simulink model "microgrid3"  (R2020a)
settings: Solver=VariableStepAuto  StartTime=0.0  StopTime=14.4  RelTol=1e-3
model workspace (MAT data in the model file):
  Sig = Simulink.Signal
  Sig.DataType = 'auto'
  Sig.Dimensions = -1
  Sig.DimensionsMode = 'auto'
  Sig.Complexity = 'auto'
  Sig.SampleTime = -1
  Sig.SamplingMode = 'auto'
libraries: powerlib x76, powerlib_meascontrol x32, eePowerMeasurement x10
settings Model: OrderedModelArguments=off  Creator=ramaz  LastModifiedBy=ramaz

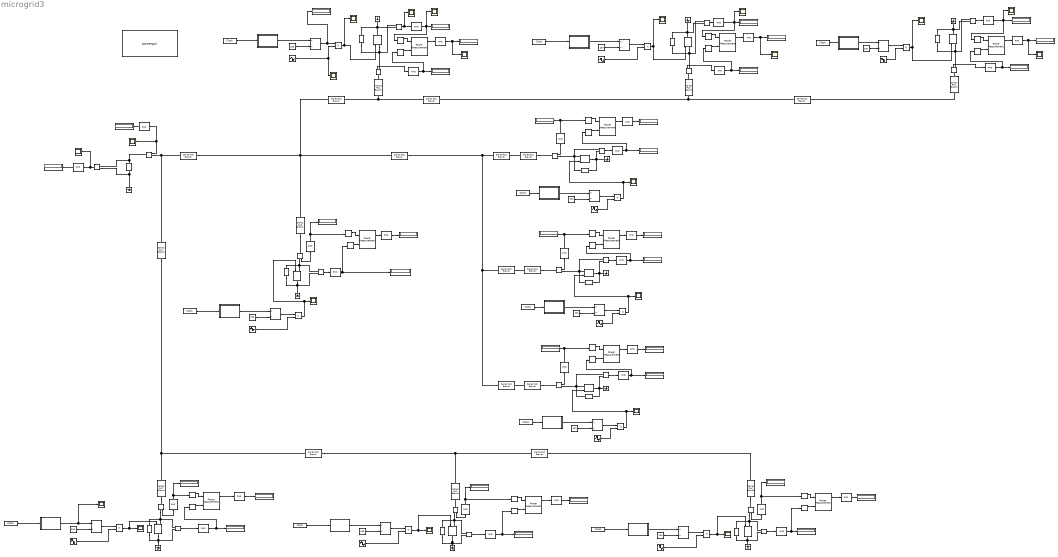
== system microgrid3 ==
  AC Voltage Source : powerlib/Electrical Sources/AC Voltage Source  Amplitude=325  Phase=0  Frequency=50  SampleTime=0  Measurements=Voltage  BusType=swing  Pref=10e3  Qref=0  Qmin=-inf  Qmax=+inf
  AMKA 16 - 45m : powerlib/Elements/Series RLC Branch  LConnTagsString=__new0  RConnTagsString=__new0  BranchType=RL  Resistance=0.08595  Inductance=1.5469860468e-5  SetiL0=off  InitialCurrent=0  Capacitance=1e-6  Setx0=off  InitialVoltage=0  Measurements=None
  AMKA 25 - 58m : powerlib/Elements/Series RLC Branch  LConnTagsString=__new0  RConnTagsString=__new0  BranchType=RL  Resistance=0.0696  Inductance=1.9569691802e-5  SetiL0=off  InitialCurrent=0  Capacitance=1e-6  Setx0=off  InitialVoltage=0  Measurements=None
  AMKA 35 - 137m : powerlib/Elements/Series RLC Branch  LConnTagsString=__new0  RConnTagsString=__new0  BranchType=RL  Resistance=0.087817  Inductance=4.4044538951e-5  SetiL0=off  InitialCurrent=0  Capacitance=1e-6  Setx0=off  InitialVoltage=0  Measurements=None
  AMKA 35 - 248m : powerlib/Elements/Series RLC Branch  LConnTagsString=__new0  RConnTagsString=__new0  BranchType=RL  Resistance=0.158968  Inductance=7.9730260291e-5  SetiL0=off  InitialCurrent=0  Capacitance=1e-6  Setx0=off  InitialVoltage=0  Measurements=None
  AMKA 35 - 33m : powerlib/Elements/Series RLC Branch  LConnTagsString=__new0  RConnTagsString=__new0  BranchType=RL  Resistance=0.021153  Inductance=1.0609268506e-5  SetiL0=off  InitialCurrent=0  Capacitance=1e-6  Setx0=off  InitialVoltage=0  Measurements=None
  AMKA 35 - 52m : powerlib/Elements/Series RLC Branch  LConnTagsString=__new0  RConnTagsString=__new0  BranchType=RL  Resistance=0.033332  Inductance=1.6717635222e-5  SetiL0=off  InitialCurrent=0  Capacitance=1e-6  Setx0=off  InitialVoltage=0  Measurements=None
  AMKA 35 - 85m : powerlib/Elements/Series RLC Branch  LConnTagsString=__new0  RConnTagsString=__new0  BranchType=RL  Resistance=0.054485  Inductance=2.8612875669e-5  SetiL0=off  InitialCurrent=0  Capacitance=1e-6  Setx0=off  InitialVoltage=0  Measurements=None
  AMKA 35 - 89m : powerlib/Elements/Series RLC Branch  LConnTagsString=__new0  RConnTagsString=__new0  BranchType=RL  Resistance=0.057049  Inductance=2.8612875669e-5  SetiL0=off  InitialCurrent=0  Capacitance=1e-6  Setx0=off  InitialVoltage=0  Measurements=None
  AMKA 35 - 95m : powerlib/Elements/Series RLC Branch  LConnTagsString=__new0  RConnTagsString=__new0  BranchType=RL  Resistance=0.060895  Inductance=3.0541833579e-5  SetiL0=off  InitialCurrent=0  Capacitance=1e-6  Setx0=off  InitialVoltage=0  Measurements=None
  AMKA 35 -89m : powerlib/Elements/Series RLC Branch  LConnTagsString=__new0  RConnTagsString=__new0  BranchType=RL  Resistance=0.03846  Inductance=1.9289579102e-5  SetiL0=off  InitialCurrent=0  Capacitance=1e-6  Setx0=off  InitialVoltage=0  Measurements=None
  AXMK 50 - 571m : powerlib/Elements/Series RLC Branch  LConnTagsString=__new0  RConnTagsString=__new0  BranchType=RL  Resistance=0.366011  Inductance=0.000159944351  SetiL0=off  InitialCurrent=0  Capacitance=1e-6  Setx0=off  InitialVoltage=0  Measurements=None
  Complex to Real-Imag{1..20} (20 alike) : ComplexToRealImag
  Constant{,1..9} (10 alike) : Constant  Value=230
  Controlled Current Source{1..10} (10 alike) : powerlib/Electrical Sources/Controlled Current Source  Initialize=on  Source_Type=AC  Amplitude=0  Phase=0  Frequency=50  Measurements=None
  Current Display : Display
  Current Display {1..11} (11 alike) : Display
  Current Measurement{,1..6,8..11} (11 alike) : powerlib/Measurements/Current Measurement  PhasorSimulation=off  OutputType=Complex  PSBequivalent=0
  Digital Clock{,1..9} (10 alike) : DigitalClock  SampleTime=0.01
  Divide{,1..9} (10 alike) : Product  Inputs=*/
  Ground{,1..10} (11 alike) : powerlib/Elements/Ground  LConnTagsString=a
  MATLAB Function : MATLAB Function  TreatAsAtomicUnit=on
  MATLAB Function1 : MATLAB Function  TreatAsAtomicUnit=on
  MATLAB Function2 : MATLAB Function  TreatAsAtomicUnit=on
  MATLAB Function3 : MATLAB Function  TreatAsAtomicUnit=on
  MATLAB Function4 : MATLAB Function  TreatAsAtomicUnit=on
  MATLAB Function5 : MATLAB Function  TreatAsAtomicUnit=on
  MATLAB Function6 : MATLAB Function  TreatAsAtomicUnit=on
  MATLAB Function7 : MATLAB Function  TreatAsAtomicUnit=on
  MATLAB Function8 : MATLAB Function  TreatAsAtomicUnit=on
  MATLAB Function9 : MATLAB Function  TreatAsAtomicUnit=on
  MC& - 40m : powerlib/Elements/Series RLC Branch  LConnTagsString=__new0  RConnTagsString=__new0  BranchType=RL  Resistance=0.1232  Inductance=1.1459155902e-5  SetiL0=off  InitialCurrent=0  Capacitance=1e-6  Setx0=off  InitialVoltage=0  Measurements=None
  MC10 - 12m : powerlib/Elements/Series RLC Branch  LConnTagsString=__new0  RConnTagsString=__new0  BranchType=RL  Resistance=0.02196  Inductance=3.3613523981e-6  SetiL0=off  InitialCurrent=0  Capacitance=1e-6  Setx0=off  InitialVoltage=0  Measurements=None
  MC10 - 29m : powerlib/Elements/Series RLC Branch  LConnTagsString=__new0  RConnTagsString=__new0  BranchType=RL  Resistance=0.06954  Inductance=1.0644282593e-6  SetiL0=off  InitialCurrent=0  Capacitance=1e-6  Setx0=off  InitialVoltage=0  Measurements=None
  MC10 - 34m : powerlib/Elements/Series RLC Branch  LConnTagsString=__new0  RConnTagsString=__new0  BranchType=RL  Resistance=0.06222  Inductance=9.5238317946e-6  SetiL0=off  InitialCurrent=0  Capacitance=1e-6  Setx0=off  InitialVoltage=0  Measurements=None
  MC10 - 35m : powerlib/Elements/Series RLC Branch  LConnTagsString=__new0  RConnTagsString=__new0  BranchType=RL  Resistance=0.06405  Inductance=9.803944944e-6  SetiL0=off  InitialCurrent=0  Capacitance=1e-6  Setx0=off  InitialVoltage=0  Measurements=None
  MC10 - 38m : powerlib/Elements/Series RLC Branch  LConnTagsString=__new0  RConnTagsString=__new0  BranchType=RL  Resistance=0.06954  Inductance=1.0644282593e-6  SetiL0=off  InitialCurrent=0  Capacitance=1e-6  Setx0=off  InitialVoltage=0  Measurements=None
  "MC10 - 38m (2) " : powerlib/Elements/Series RLC Branch  LConnTagsString=__new0  RConnTagsString=__new0  BranchType=RL  Resistance=0.06954  Inductance=1.0644282593e-5  SetiL0=off  InitialCurrent=0  Capacitance=1e-6  Setx0=off  InitialVoltage=0  Measurements=None
  MC10 - 48m : powerlib/Elements/Series RLC Branch  LConnTagsString=__new0  RConnTagsString=__new0  BranchType=RL  Resistance=0.08784  Inductance=1.3502705371e-5  SetiL0=off  InitialCurrent=0  Capacitance=1e-6  Setx0=off  InitialVoltage=0  Measurements=None
  MC6 - 11m : powerlib/Elements/Series RLC Branch  LConnTagsString=__new0  RConnTagsString=__new0  BranchType=RL  Resistance=0.03388  Inductance=3.1512678737e-6  SetiL0=off  InitialCurrent=0  Capacitance=1e-6  Setx0=off  InitialVoltage=0  Measurements=None
  MC6 - 4m : powerlib/Elements/Series RLC Branch  LConnTagsString=__new0  RConnTagsString=__new0  BranchType=RL  Resistance=0.01232  Inductance=1.1459155902e-6  SetiL0=off  InitialCurrent=0  Capacitance=1e-6  Setx0=off  InitialVoltage=0  Measurements=None
  Power Measurement1 : eePowerMeasurement/Power Measurement  LabelModeActiveChoice=Continuous  F=50  K=[0]  Ts=0
      settings: SourceProductBaseCode=PS
  Power Measurement10 : eePowerMeasurement/Power Measurement  LabelModeActiveChoice=Continuous  F=50  K=[0]  Ts=0
      settings: SourceProductBaseCode=PS
  Power Measurement2 : eePowerMeasurement/Power Measurement  LabelModeActiveChoice=Continuous  F=50  K=[0]  Ts=0
      settings: SourceProductBaseCode=PS
  Power Measurement{3..9} (7 alike) : eePowerMeasurement/Power Measurement  LabelModeActiveChoice=Continuous  F=60  K=[0]  Ts=0
      settings: SourceProductBaseCode=PS
  Power Display {1..10} (10 alike) : Display
  Product{,1..9} (10 alike) : Product
  RMS{1..32} (32 alike) : powerlib_meascontrol/Measurements/RMS  TrueRMS=on  Freq=50  RMSInit=0  Ts=0
  Scope{1..21} (21 alike) : Scope
  Series RLC Branch{18..27} (10 alike) : powerlib/Elements/Series RLC Branch  LConnTagsString=__new0  RConnTagsString=__new0  BranchType=R  Resistance=100000000  Inductance=1e-3  SetiL0=off  InitialCurrent=0  Capacitance=1e-6  Setx0=off  InitialVoltage=0  Measurements=None
  Sine Wave{,1..9} (10 alike) : Sin  Frequency=50  SampleTime=0
  Voltage Display : Display
  Voltage Display {1..10} (10 alike) : Display
  Voltage Measurement{,1..4,6..9,11} (10 alike) : powerlib/Measurements/Voltage Measurement  PhasorSimulation=off  OutputType=Complex  PSBequivalent=0
  Voltage Measurement10 : powerlib/Measurements/Voltage Measurement  PhasorSimulation=off  OutputType=Magnitude  PSBequivalent=0
  powergui : powerlib/powergui  Priority=1  SimulationMode=Discrete  SampleTime=5e-5  frequency=50  Iterations=50  frequencyindice=50  Pbase=100e6  ErrMax=1e-4  UnitsV=kV  UnitsW=MW  buscounter=0  FunctionMessages=off  echomessages=off  EnableUseOfTLC=off  CurrentSourceSwitches=off  DisableSnubberDevices=off  DisableRonSwitches=off  DisableVfSwitches=off  DisplayEquations=off  AutomaticDiscreteSolvers=off  SolverType=Tustin/Backward Euler (TBE)  Interpol=off  ExternalGateDelay=off  methode=off  Ts=100  x0status=blocks  SPID=on  SwTol=0  HookPort=off  NonlinearTolerance=1e-4  nMaxIteration=100  ContinueOnMaxIteration=off  RestoreLinks=warning  ResistiveCurrentMeasurement=off  Frange=[0:2:500]  Ylog=off  Xlog=on  ShowGrid=off  save=off  variable=ZData  structure=0  ZoomFFT=off  StartTime=0.0  cycles=1  DisplayStyle=1  fundamental=60  FreqAxis=off  MaxFrequency=1000  frequencyindicesteady=1  RmsSteady=1  display=off
  wires:
  Current Measurement/1 -> RMS3/1
  Voltage Measurement/1 -> Scope21/1, RMS1/1
  Current Measurement3/1 -> RMS9/1
  Current Measurement4/1 -> RMS10/1
  Current Measurement5/1 -> RMS13/1
  Voltage Measurement3/1 -> RMS8/1
  Voltage Measurement4/1 -> RMS11/1
  Voltage Measurement11/1 -> RMS12/1
  Voltage Measurement6/1 -> RMS23/1
  Current Measurement8/1 -> RMS24/1
  Current Measurement9/1 -> RMS19/1
  Voltage Measurement8/1 -> RMS18/1
  Current Measurement10/1 -> RMS17/1
  Voltage Measurement7/1 -> RMS16/1
  Voltage Measurement9/1 -> RMS14/1
  Current Measurement11/1 -> RMS15/1
  Complex to Real-Imag4/1 -> Power Measurement2/2
  Complex to Real-Imag5/1 -> Power Measurement2/1
  Power Measurement2/1 -> RMS20/1
  Complex to Real-Imag6/1 -> Power Measurement3/2
  Complex to Real-Imag7/1 -> Power Measurement3/1
  Power Measurement3/1 -> RMS27/1
  Complex to Real-Imag8/1 -> Power Measurement4/2
  Complex to Real-Imag9/1 -> Power Measurement4/1
  Power Measurement4/1 -> RMS26/1
  Complex to Real-Imag10/1 -> Power Measurement5/2
  Complex to Real-Imag11/1 -> Power Measurement5/1
  Power Measurement5/1 -> RMS28/1
  Complex to Real-Imag12/1 -> Power Measurement6/2
  Complex to Real-Imag13/1 -> Power Measurement6/1
  Complex to Real-Imag14/1 -> Power Measurement7/2
  Complex to Real-Imag15/1 -> Power Measurement7/1
  Power Measurement7/1 -> RMS31/1
  Complex to Real-Imag16/1 -> Power Measurement8/2
  Complex to Real-Imag17/1 -> Power Measurement8/1
  Power Measurement8/1 -> RMS30/1
  Complex to Real-Imag18/1 -> Power Measurement9/2
  Complex to Real-Imag19/1 -> Power Measurement9/1
  Power Measurement9/1 -> RMS29/1
  RMS1/1 -> Scope1/1, Voltage Display 1/1, Complex to Real-Imag5/1
  RMS3/1 -> Complex to Real-Imag4/1, Current Display 1/1
  RMS5/1 -> Complex to Real-Imag2/1, Current Display 2/1
  Complex to Real-Imag2/1 -> Power Measurement1/2
  Power Measurement1/1 -> RMS21/1
  RMS4/1 -> Scope5/1, Voltage Display 2/1, Complex to Real-Imag3/1
  Complex to Real-Imag3/1 -> Power Measurement1/1
  Current Measurement1/1 -> RMS5/1
  Voltage Measurement1/1 -> RMS4/1
  Complex to Real-Imag20/1 -> Power Measurement10/1
  Power Measurement10/1 -> RMS22/1
  Complex to Real-Imag1/1 -> Power Measurement10/2
  RMS6/1 -> Complex to Real-Imag20/1, Voltage Display 3/1, Scope7/1
  Voltage Measurement2/1 -> RMS6/1
  RMS7/1 -> Complex to Real-Imag1/1, Current Display 3/1
  Current Measurement2/1 -> RMS7/1
  RMS8/1 -> Voltage Display 5/1, Complex to Real-Imag6/1
  RMS9/1 -> Current Display 5/1, Complex to Real-Imag7/1
  RMS10/1 -> Current Display 6/1, Complex to Real-Imag9/1
  RMS11/1 -> Voltage Display 6/1, Complex to Real-Imag8/1
  RMS12/1 -> Voltage Display 7/1, Complex to Real-Imag10/1
  RMS13/1 -> Current Display 7/1, Complex to Real-Imag11/1
  RMS14/1 -> Complex to Real-Imag18/1, Voltage Display 10/1
  RMS15/1 -> Complex to Real-Imag19/1, Current Display 10/1
  RMS16/1 -> Complex to Real-Imag16/1, Voltage Display 9/1
  RMS17/1 -> Complex to Real-Imag17/1, Current Display 9/1
  RMS18/1 -> Complex to Real-Imag14/1, Voltage Display 8/1
  RMS19/1 -> Complex to Real-Imag15/1, Current Display 8/1
  RMS20/1 -> Power Display 1/1, Scope4/1
  RMS21/1 -> Power Display 2/1, Scope6/1
  RMS22/1 -> Power Display 3/1, Scope8/1
  RMS23/1 -> Voltage Display 4/1, Complex to Real-Imag12/1
  RMS24/1 -> Current Display 4/1, Complex to Real-Imag13/1
  Power Measurement6/1 -> RMS25/1
  RMS25/1 -> Power Display 4/1
  RMS26/1 -> Power Display 6/1
  RMS27/1 -> Power Display 5/1
  RMS28/1 -> Power Display 7/1
  RMS30/1 -> Power Display 9/1
  RMS31/1 -> Power Display 8/1
  RMS29/1 -> Power Display 10/1
  Current Measurement6/1 -> RMS32/1, Scope3/1
  RMS32/1 -> Current Display/1
  Voltage Measurement10/1 -> Scope2/1, RMS2/1
  RMS2/1 -> Voltage Display/1
  MATLAB Function/1(y) -> Divide/1
  Digital Clock/1 -> MATLAB Function/1(time)
  Sine Wave/1 -> Scope20/1, Product/2
  Constant/1 -> Divide/2
  Divide/1 -> Current Display 11/1, Product/1
  Product/1 -> Scope9/1, Controlled Current Source1/1
  Product1/1 -> Controlled Current Source2/1, Scope10/1
  Divide1/1 -> Product1/1
  Digital Clock1/1 -> MATLAB Function1/1(time)
  MATLAB Function1/1(y) -> Divide1/1
  Constant1/1 -> Divide1/2
  Sine Wave1/1 -> Product1/2
  Divide2/1 -> Product2/1
  Constant2/1 -> Divide2/2
  Digital Clock2/1 -> MATLAB Function2/1(time)
  Sine Wave2/1 -> Product2/2
  Product2/1 -> Controlled Current Source3/1, Scope11/1
  MATLAB Function2/1(y) -> Divide2/1
  Divide3/1 -> Product3/1
  Constant3/1 -> Divide3/2
  Digital Clock3/1 -> MATLAB Function3/1(time)
  Sine Wave3/1 -> Product3/2
  Product3/1 -> Scope12/1, Controlled Current Source5/1
  MATLAB Function3/1(y) -> Divide3/1
  Divide4/1 -> Product4/1
  Digital Clock4/1 -> MATLAB Function4/1(time)
  Sine Wave4/1 -> Product4/2
  Constant4/1 -> Divide4/2
  MATLAB Function4/1(y) -> Divide4/1
  Product4/1 -> Controlled Current Source6/1, Scope13/1
  Product5/1 -> Controlled Current Source7/1, Scope14/1
  MATLAB Function5/1(y) -> Divide5/1
  Sine Wave5/1 -> Product5/2
  Divide5/1 -> Product5/1
  Digital Clock5/1 -> MATLAB Function5/1(time)
  Constant5/1 -> Divide5/2
  Product6/1 -> Scope15/1, Controlled Current Source4/1
  Divide6/1 -> Product6/1
  Digital Clock6/1 -> MATLAB Function6/1(time)
  MATLAB Function6/1(y) -> Divide6/1
  Constant6/1 -> Divide6/2
  Sine Wave6/1 -> Product6/2
  Constant7/1 -> Divide7/2
  Sine Wave7/1 -> Product7/2
  Digital Clock7/1 -> MATLAB Function7/1(time)
  Product7/1 -> Scope16/1, Controlled Current Source8/1
  Divide7/1 -> Product7/1
  MATLAB Function7/1(y) -> Scope19/1, Divide7/1
  Product8/1 -> Controlled Current Source9/1, Scope17/1
  Digital Clock8/1 -> MATLAB Function8/1(time)
  Divide8/1 -> Product8/1
  Constant8/1 -> Divide8/2
  Sine Wave8/1 -> Product8/2
  MATLAB Function8/1(y) -> Divide8/1
  Product9/1 -> Controlled Current Source10/1, Scope18/1
  Digital Clock9/1 -> MATLAB Function9/1(time)
  Divide9/1 -> Product9/1
  Constant9/1 -> Divide9/2
  Sine Wave9/1 -> Product9/2
  MATLAB Function9/1(y) -> Divide9/1
  connections:
  AC Voltage Source/LConn1 -- Voltage Measurement10/LConn2 -- Ground/LConn1
  AMKA 35 - 85m/LConn1 -- Current Measurement6/RConn1 -- AMKA 35 - 89m/LConn1
  Current Measurement8/RConn1 -- Series RLC Branch21/LConn1 -- Controlled Current Source4/LConn1 -- Voltage Measurement6/LConn1
  Voltage Measurement4/LConn1 -- Controlled Current Source6/LConn1 -- Current Measurement4/RConn1 -- Series RLC Branch23/LConn1
  Series RLC Branch24/LConn1 -- Voltage Measurement3/LConn1 -- Controlled Current Source5/LConn1 -- Current Measurement3/RConn1
  Current Measurement5/RConn1 -- Voltage Measurement11/LConn1 -- Controlled Current Source7/LConn1 -- Series RLC Branch22/LConn1
  MC10 - 48m/LConn1 -- AMKA 35 - 95m/LConn1 -- AMKA 35 -89m/RConn1
  Current Measurement/RConn1 -- Voltage Measurement/LConn1 -- Controlled Current Source1/LConn1 -- Series RLC Branch27/RConn1
  Current Measurement1/RConn1 -- Voltage Measurement1/LConn1 -- Controlled Current Source2/LConn1 -- Series RLC Branch26/RConn1
  Current Measurement2/RConn1 -- Series RLC Branch25/LConn1 -- Voltage Measurement2/LConn1 -- Controlled Current Source3/LConn1
  AMKA 35 - 248m/RConn1 -- AMKA 35 - 137m/LConn1 -- AMKA 35 - 33m/LConn1 -- AMKA 16 - 45m/LConn1
  AMKA 35 - 89m/RConn1 -- AMKA 35 -89m/LConn1 -- AMKA 35 - 248m/LConn1 -- MC10 - 38m/LConn1
  Current Measurement9/RConn1 -- Voltage Measurement8/LConn1 -- Controlled Current Source8/LConn1 -- Series RLC Branch18/LConn1
  AMKA 35 - 85m/RConn1 -- AMKA 35 - 52m/LConn1 -- MC10 - 29m/LConn1
  AMKA 35 - 52m/RConn1 -- MC10 - 35m/LConn1 -- AMKA 25 - 58m/LConn1
  Current Measurement10/RConn1 -- Voltage Measurement7/LConn1 -- Controlled Current Source9/LConn1 -- Series RLC Branch19/LConn1
  Current Measurement11/RConn1 -- Series RLC Branch20/LConn1 -- Controlled Current Source10/LConn1 -- Voltage Measurement9/LConn1
  Ground1/LConn1 -- Voltage Measurement8/LConn2 -- Controlled Current Source8/RConn1 -- Series RLC Branch18/RConn1
  Voltage Measurement7/LConn2 -- Ground2/LConn1 -- Controlled Current Source9/RConn1 -- Series RLC Branch19/RConn1
  Voltage Measurement9/LConn2 -- Controlled Current Source10/RConn1 -- Series RLC Branch20/RConn1 -- Ground3/LConn1
  Voltage Measurement11/LConn2 -- Series RLC Branch22/RConn1 -- Controlled Current Source7/RConn1 -- Ground4/LConn1
  Voltage Measurement4/LConn2 -- Series RLC Branch23/RConn1 -- Controlled Current Source6/RConn1 -- Ground5/LConn1
  Voltage Measurement3/LConn2 -- Ground6/LConn1 -- Controlled Current Source5/RConn1 -- Series RLC Branch24/RConn1
  Voltage Measurement2/LConn2 -- Controlled Current Source3/RConn1 -- Series RLC Branch25/RConn1 -- Ground7/LConn1
  Ground8/LConn1 -- Controlled Current Source2/RConn1 -- Voltage Measurement1/LConn2 -- Series RLC Branch26/LConn1
  Series RLC Branch21/RConn1 -- Voltage Measurement6/LConn2 -- Controlled Current Source4/RConn1 -- Ground10/LConn1
  MC10 - 48m/RConn1 -- Current Measurement/LConn1
  MC10 - 34m/RConn1 -- Current Measurement1/LConn1
  MC6 - 4m/RConn1 -- Current Measurement2/LConn1
  MC6 - 11m/LConn1 -- AMKA 16 - 45m/RConn1
  MC6 - 11m/RConn1 -- Current Measurement3/LConn1
  AMKA 35 - 137m/RConn1 -- MC10 - 12m/LConn1
  MC10 - 12m/RConn1 -- Current Measurement4/LConn1
  AMKA 35 - 33m/RConn1 -- "MC10 - 38m (2) "/LConn1
  "MC10 - 38m (2) "/RConn1 -- Current Measurement5/LConn1
  MC10 - 38m/RConn1 -- Current Measurement8/LConn1
  MC10 - 29m/RConn1 -- Current Measurement9/LConn1
  Current Measurement10/LConn1 -- MC10 - 35m/RConn1
  MC& - 40m/RConn1 -- Current Measurement11/LConn1
  AMKA 25 - 58m/RConn1 -- MC& - 40m/LConn1
  AXMK 50 - 571m/RConn1 -- MC6 - 4m/LConn1
  MC10 - 34m/LConn1 -- AMKA 35 - 95m/RConn1 -- AXMK 50 - 571m/LConn1
  AC Voltage Source/RConn1 -- Current Measurement6/LConn1 -- Voltage Measurement10/LConn1
  Voltage Measurement/LConn2 -- Series RLC Branch27/LConn1 -- Ground9/LConn1 -- Controlled Current Source1/RConn1

== matlab function microgrid3/MATLAB Function ==
  data: time input; y output
function y = fcn(time)
    file = fopen('C:\\Users\\ramaz\\Desktop\\Bitirme_Projesi\\microgrid_matlab\\house1\\house_1_consume_power_1.txt','r');
    formatSpec = '%d';
    x = fscanf(file,formatSpec);
    time = time*100;
    if time == 0
        y = 0;
    elseif floor(time) == time
        y = x(time);
    else
        if floor(time) ~= 0
            y = x(floor(time));
        else
            y = 0;
        end
    end
    fclose(file);
end

== matlab function microgrid3/MATLAB Function2 ==
  data: time input; y output
function y = fcn(time)
    file = fopen('C:\\Users\\ramaz\\Desktop\\Bitirme_Projesi\\microgrid_matlab\\house3\\house_3_consume_power_1.txt','r');
    formatSpec = '%d';
    x = fscanf(file,formatSpec);
    time = time*100;
    if time == 0
        y = 0;
    elseif floor(time) == time
        y = x(time);
    else
        if floor(time) ~= 0
            y = x(floor(time));
        else
            y = 0;
        end
    end
    fclose(file);
end

== matlab function microgrid3/MATLAB Function3 ==
  data: time input; y output
function y = fcn(time)
    file = fopen('C:\\Users\\ramaz\\Desktop\\Bitirme_Projesi\\microgrid_matlab\\house5\\house_5_consume_power_1.txt','r');
    formatSpec = '%d';
    x = fscanf(file,formatSpec);
    time = time*100;
    if time == 0
        y = 0;
    elseif floor(time) == time
        y = x(time);
    else
        if floor(time) ~= 0
            y = x(floor(time));
        else
            y = 0;
        end
    end
    fclose(file);
end

== matlab function microgrid3/MATLAB Function4 ==
  data: time input; y output
function y = fcn(time)
    file = fopen('C:\\Users\\ramaz\\Desktop\\Bitirme_Projesi\\microgrid_matlab\\house6\\house_6_consume_power_1.txt','r');
    formatSpec = '%d';
    x = fscanf(file,formatSpec);
    time = time*100;
    if time == 0
        y = 0;
    elseif floor(time) == time
        y = x(time);
    else
        if floor(time) ~= 0
            y = x(floor(time));
        else
            y = 0;
        end
    end
    fclose(file);
end

== matlab function microgrid3/MATLAB Function5 ==
  data: time input; y output
function y = fcn(time)
    file = fopen('C:\\Users\\ramaz\\Desktop\\Bitirme_Projesi\\microgrid_matlab\\house7\\house_7_consume_power_1.txt','r');
    formatSpec = '%d';
    x = fscanf(file,formatSpec);
    time = time*100;
    if time == 0
        y = 0;
    elseif floor(time) == time
        y = x(time);
    else
        if floor(time) ~= 0
            y = x(floor(time));
        else
            y = 0;
        end
    end
    fclose(file);
end

== matlab function microgrid3/MATLAB Function6 ==
  data: time input; y output
function y = fcn(time)
    file = fopen('C:\\Users\\ramaz\\Desktop\\Bitirme_Projesi\\microgrid_matlab\\house4\\house_4_consume_power_1.txt','r');
    formatSpec = '%d';
    x = fscanf(file,formatSpec);
    time = time*100;
    if time == 0
        y = 0;
    elseif floor(time) == time
        y = x(time);
    else
        if floor(time) ~= 0
            y = x(floor(time));
        else
            y = 0;
        end
    end
    fclose(file);
end

== matlab function microgrid3/MATLAB Function7 ==
  data: time input; y output
function y = fcn(time)
    file = fopen('C:\\Users\\ramaz\\Desktop\\Bitirme_Projesi\\microgrid_matlab\\house8\\house_8_consume_power_1.txt','r');
    formatSpec = '%d';
    x = fscanf(file,formatSpec);
    time = time*100;
    if time == 0
        y = 0;
    elseif floor(time) == time
        y = x(time);
    else
        if floor(time) ~= 0
            y = x(floor(time));
        else
            y = 0;
        end
    end
    fclose(file);
end

== matlab function microgrid3/MATLAB Function8 ==
  data: time input; y output
function y = fcn(time)
    file = fopen('C:\\Users\\ramaz\\Desktop\\Bitirme_Projesi\\microgrid_matlab\\house9\\house_9_consume_power_1.txt','r');
    formatSpec = '%d';
    x = fscanf(file,formatSpec);
    time = time*100;
    if time == 0
        y = 0;
    elseif floor(time) == time
        y = x(time);
    else
        if floor(time) ~= 0
            y = x(floor(time));
        else
            y = 0;
        end
    end
    fclose(file);
end

== matlab function microgrid3/MATLAB Function9 ==
  data: time input; y output
function y = fcn(time)
    file = fopen('C:\\Users\\ramaz\\Desktop\\Bitirme_Projesi\\microgrid_matlab\\house10\\house_10_consume_power_1.txt','r');
    formatSpec = '%d';
    x = fscanf(file,formatSpec);
    time = time*100;
    if time == 0
        y = 0;
    elseif floor(time) == time
        y = x(time);
    else
        if floor(time) ~= 0
            y = x(floor(time));
        else
            y = 0;
        end
    end
    fclose(file);
end

== matlab function microgrid3/MATLAB Function1 ==
  data: time input; y output
function y = fcn(time)
    file = fopen('C:\\Users\\ramaz\\Desktop\\Bitirme_Projesi\\microgrid_matlab\\house2\\house_2_consume_power_1.txt','r');
    formatSpec = '%d';
    x = fscanf(file,formatSpec);
    time = time*100;
    if time == 0
        y = 0;
    elseif floor(time) == time
        y = x(time);
    else
        if floor(time) ~= 0
            y = x(floor(time));
        else
            y = 0;
        end
    end
    fclose(file);
end
